simulink model "linmod_model_MIMO"  (R2018b)
settings: Solver=VariableStepAuto  StartTime=0.0  StopTime=10.0  RelTol=1e-3
undefined symbols (not defined in the file or in its folder): GEOMETRY
libraries: PlanarVehicle x2
settings Model: Creator=Christopher  LastModifiedBy=Christopher
settings DataIOCC: ExternalInput=getinputstruct(op_trim)  InitialState=getstatestruct(op_trim)

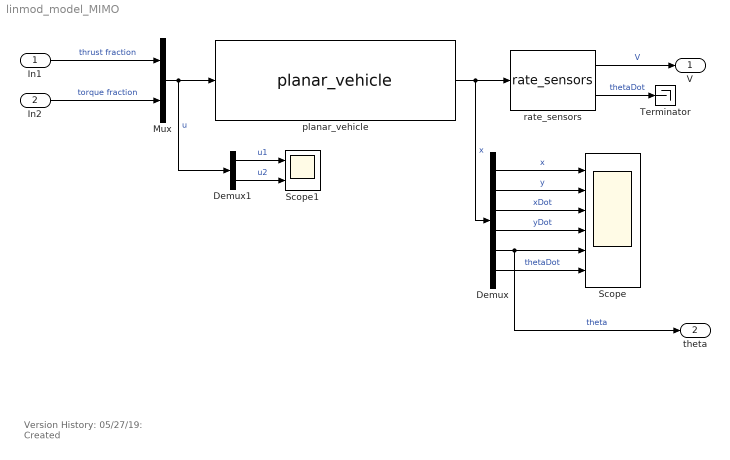
== system linmod_model_MIMO ==
  note: Version History:
      | 05/27/19: Created
  In1 : Inport
  In2 : Inport  Port=2
  Demux : Demux  Outputs=6
  Demux1 : Demux  Outputs=2
  Mux : Mux  Inputs=2
  Scope : Scope  NumInputPorts=6
  Scope1 : Scope  NumInputPorts=2
  Terminator : Terminator
  planar_vehicle : PlanarVehicle/planar_vehicle  m=GEOMETRY.mass  Ib=GEOMETRY.Ib  Fmax=PROPULSION.Fmax  Mmax=PROPULSION.Mmax  x0=SIMULATION.X_0  CT=ENVIRONMENT.CT  CR=ENVIRONMENT.CR
  rate_sensors : PlanarVehicle/rate_sensors
  V : Outport
  theta : Outport  Port=2
  wires:
  In2/1 -> Mux/2  "torque fraction"
  Mux/1 -> Demux1/1, planar_vehicle/1  "u"
  planar_vehicle/1 -> rate_sensors/1, Demux/1  "x"
  Demux/4 -> Scope/4  "yDot"
  Demux/3 -> Scope/3  "xDot"
  Demux/5 -> theta/1, Scope/5  "theta"
  Demux/2 -> Scope/2  "y"
  Demux/6 -> Scope/6  "thetaDot"
  Demux/1 -> Scope/1  "x"
  Demux1/1 -> Scope1/1  "u1"
  Demux1/2 -> Scope1/2  "u2"
  rate_sensors/1 -> V/1  "V"
  rate_sensors/2 -> Terminator/1  "thetaDot"
  In1/1 -> Mux/1  "thrust fraction"
